simulink model "SimCompleta"  (R2022a)
settings: Solver=VariableStepAuto  StartTime=0.0  StopTime=10.0  RelTol=1e-3
values from neighbouring files (symbols this model uses):
  vo = 0.1    [Parametros.m]
  xa = 39.5/1000    (= 0.0395)    [Parametros.m]
undefined symbols (not defined in the file or in its folder): theta0, wo
libraries: cstblocks x1
settings Model: Creator=Francisco  LastModifiedBy=Francisco

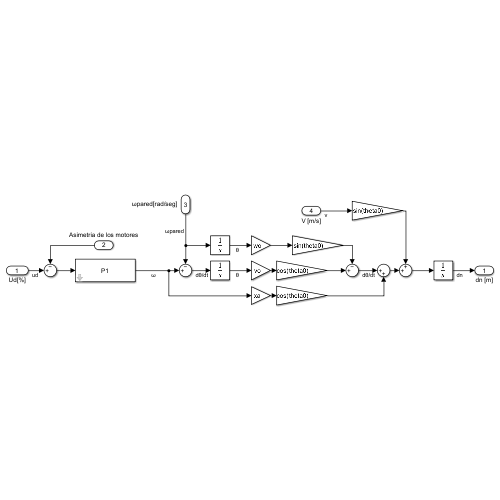
[thumbnail: Simulink's stored preview of the top-level diagram]
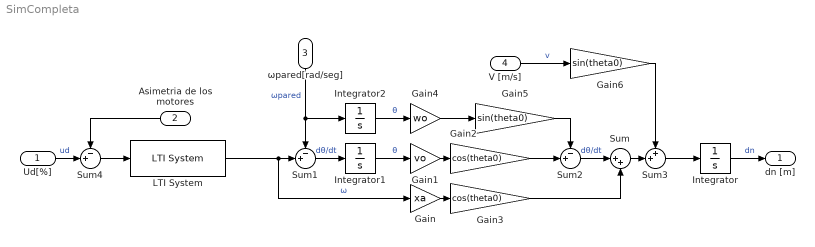
== system SimCompleta ==
  Ud[%] : Inport
  Asimetria de los motores : Inport  Port=2
  ωpared[rad/seg] : Inport  Port=3
  V [m/s] : Inport  Port=4
  Gain : Gain  Gain=xa
  Gain1 : Gain  Gain=vo
  Gain2 : Gain  Gain=cos(theta0)
  Gain3 : Gain  Gain=cos(theta0)
  Gain4 : Gain  Gain=wo
  Gain5 : Gain  Gain=sin(theta0)
  Gain6 : Gain  Gain=sin(theta0)
  Integrator : Integrator
  Integrator1 : Integrator
  Integrator2 : Integrator
  LTI System : cstblocks/LTI System  sys=P1  IC=[]
  Sum : Sum  Inputs=|++
  Sum1 : Sum  Inputs=-+|
  Sum2 : Sum  Inputs=-+|
  Sum3 : Sum  Inputs=++|
  Sum4 : Sum  Inputs=-+|
  dn [m] : Outport
  wires:
  LTI System/1 -> Sum1/2, Gain/1  "ω"
  Integrator1/1 -> Gain1/1  "θ"
  Gain/1 -> Gain3/1
  Sum1/1 -> Integrator1/1  "dθ/dt"
  Gain1/1 -> Gain2/1
  ωpared[rad/seg]/1 -> Integrator2/1, Sum1/1  "ωpared"
  Integrator/1 -> dn [m]/1  "dn"
  Gain3/1 -> Sum/2
  Gain4/1 -> Gain5/1
  Integrator2/1 -> Gain4/1  "θ"
  Sum2/1 -> Sum/1  "dθ/dt"
  Gain2/1 -> Sum2/2
  Gain5/1 -> Sum2/1
  Sum3/1 -> Integrator/1
  Sum/1 -> Sum3/2
  Gain6/1 -> Sum3/1
  V [m/s]/1 -> Gain6/1  "v"
  Asimetria de los motores/1 -> Sum4/1
  Ud[%]/1 -> Sum4/2  "ud"
  Sum4/1 -> LTI System/1
